simulink model "test_bench"  (Simulink 9.2)
settings: Solver=FixedStepDiscrete  StartTime=0.0  StopTime=inf  FixedStep=t_sample_s  RelTol=1e-3
values from neighbouring files (symbols this model uses):
  f_tp_Hz = 1    [init.m]
  I_gain = [4,4,8,6,11]*1e-2*1    [init.m]
  mpc_flag = 0    [init.m]
  n_akt = 5    [init.m]    (also in postprocess.m)
  offset_q_offline = [266.1,185.3,200.5,240.7,168.1]    [init.m]
  P_gain = [4,6,11,11,10]*1e-2*1    [init.m]
  p_max_bar = 0.7    [init.m]
  pi_flag = 1    [init.m]
  t_sample_s = 1e-3    (= 0.001)    [init.m]
libraries: test_bench_lib x23, etherlab_lib x10, simulink x5, dspsigops x2, pePwmGenerator x1
settings Model: Creator=moritz  LastModifiedBy=entwicklungs-pc  SimulationMode=external  ExtModeTrigDuration=10000  ExtModeArchiveMode=auto  ExtModeArchiveFileName=measurement_data  ExtModeArchiveDirName=./results  ExtModeLogAll=off
settings DataIOCC: LimitDataPoints=off  SaveFormat=Dataset  SignalLoggingSaveFormat=Dataset  SaveOutput=off  SignalLogging=off  SaveTime=off
settings OptimizationCC: BlockReduction=off  ConditionallyExecuteInputs=off  OptimizeBlockIOStorage=off  BufferReuse=off  GlobalBufferReuse=off  ExpressionFolding=off  LocalBlockOutputs=off  LifeSpan=auto  OptimizeDataStoreBuffers=off  BusAssignmentInplaceUpdate=off
settings DebuggingCC: UnderspecifiedInitializationDetection=Simplified  MergeDetectMultiDrivingBlocksExec=error  FcnCallInpInsideContextMsg=error  StateNameClashWarn=none  SFUnexpectedBacktrackingDiag=error  SFNoUnconditionalDefaultTransitionDiag=error  SFExecutionAtInitializationDiag=warning
settings HardwareCC: ProdBitPerPointer=64  ProdBitPerSizeT=64  ProdBitPerPtrDiffT=64  ProdLargestAtomicFloat=Float  ProdIntDivRoundTo=Zero  ProdEndianess=LittleEndian  ProdWordSize=64  ProdHWDeviceType=Intel->x86-64 (Windows64)
settings ModelReferenceCC: PropagateSignalLabelsOutOfModel=on
settings RTWCC: SystemTargetFile=etherlab.tlc  TemplateMakefile=etherlab_hrt.tmf  Description=EtherLab PREEMT_RT Real-Time Target
settings CodeAppCC: StateflowObjectComments=off
settings STFCustomTargetCC: TargetLangStandard=C99 (ISO)  ModelReferenceCompliant=off  SystemTargetFile=etherlab.tlc
settings GRTTargetCC: TargetLangStandard=C99 (ISO)  ModelReferenceCompliant=off  ParMdlRefBuildCompliant=off  CompOptLevelCompliant=off  ConcurrentExecutionCompliant=off  GeneratePreprocessorConditionals=Use local settings  MatFileLogging=off  CPPClassGenCompliant=off  UseToolchainInfoCompliant=off  ExtMode=on  ExtModeStaticAlloc=on  ExtModeStaticAllocSize=50000000  ExtModeMexArgs='130.75.144.164' 0 17725  RTWCAPISignals=on  RTWCAPIParams=on
settings CustomProperty: DataType=int32  Value=2
settings ConfigComp: CovMetricSettings=dwe  CovHtmlReporting=off  CovSaveCumulativeToWorkspaceVar=off  CovSaveSingleToWorkspaceVar=off  CovExternalEMLEnable=on

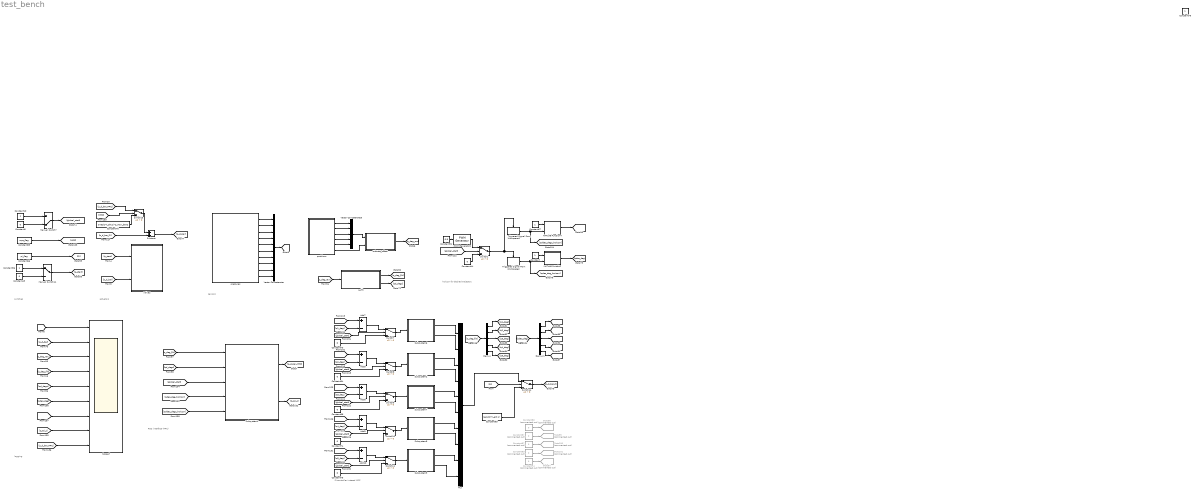
== system test_bench ==
  note: sensors
  note: actuators
  note: logging
  note: switches
  note: ROS interface (MPC)
  note: horizon for desired trajectory
  note: PI-controller instead MPC
  Add{5,7..10} (5 alike) : Sum  Inputs=+-
  Constant{,10,36,67} (4 alike) : Constant  SampleTime=t_sample_s
  Constant{5,43,64,68,73..75} (7 alike) : Constant  Value=0  SampleTime=t_sample_s
  Constant44 : Constant  Value=0  SampleTime=1e-3
  Constant51 : Constant  Value=0.5  SampleTime=t_sample_s
  Constant65 : Constant  Value=zeros(2*n_akt,1)  SampleTime=t_sample_s
  Constant66 : Constant  Value=pi_flag  SampleTime=t_sample_s
  Constant76 : Constant  Value=ones(2*n_akt,1)*p_max_bar/2  SampleTime=t_sample_s
  Constant78 : Constant
  Constant{80..84} (5 alike) : Constant  Commented=on  Value=0
  Constant85 : Constant  Value=mpc_flag  SampleTime=t_sample_s
  Demux : Demux  Outputs=5
  Demux1 : Demux  Outputs=5
  Goto100 : Goto  Commented=on  GotoTag=q3des_deg
  Goto101 : Goto  Commented=on  GotoTag=q4des_deg
  Goto97 : Goto  Commented=on  GotoTag=q5des_deg
  Goto98 : Goto  Commented=on  GotoTag=q1des_deg
  Goto99 : Goto  Commented=on  GotoTag=q2des_deg
  MATLAB Function : MATLAB Function  TreatAsAtomicUnit=on
  MATLAB Function4 : MATLAB Function  TreatAsAtomicUnit=on
  Manual Switch11 : ManualSwitch
  Manual Switch7 : ManualSwitch  CurrentSetting=0
  Mux : Mux  Inputs=10
  PWM Generator2 : pePwmGenerator/PWM Generator  CarrCount=Up  Tper=t_sample_MPC_s  Ts=t_sample_s
  Scope7 : Scope  NumInputPorts=9
  Subsystem2 : Subsystem
  Subsystem4 : Subsystem
  Subsystem6 : Subsystem
  Subsystem7 : Subsystem
  Subsystem8 : Subsystem
  Subsystem9 : Subsystem
  Subtract : Sum
  Switch{1,7..11,13..14} (8 alike) : Switch  Criteria=u2 > Threshold
  Triggered Signal From Workspace1 : dspsigops/Triggered Signal From Workspace  Signal=Qd_total  TriggerType=Rising edge  ic=0  SamplesPerFrame=1  OutputAfterFinalValue=Setting to zero  OutputFrames=off
      settings: SourceProductName=DSP System Toolbox  SourceProductBaseCode=DS
  Triggered Signal From Workspace2 : dspsigops/Triggered Signal From Workspace  Signal=Q_total  TriggerType=Rising edge  ic=0  SamplesPerFrame=1  OutputAfterFinalValue=Setting to zero  OutputFrames=off
      settings: SourceProductName=DSP System Toolbox  SourceProductBaseCode=DS
  Vector Concatenate : Concatenate  NumInputs=10
  Vector Concatenate3 : Concatenate  NumInputs=5
  positions : Subsystem
  pressures : Subsystem
  q_filt : Subsystem
  subtract_offset : MATLAB Function  TreatAsAtomicUnit=on
  "valves " : Subsystem
  wires:
  pressures/3("p21_bar ") -> Vector Concatenate/3
  pressures/4(p22_bar) -> Vector Concatenate/4
  pressures/1("p11_bar ") -> Vector Concatenate/1
  pressures/2(p12_bar) -> Vector Concatenate/2
  pressures/5(p31_bar) -> Vector Concatenate/5
  pressures/6(p32_bar) -> Vector Concatenate/6
  pressures/7(p41_bar) -> Vector Concatenate/7
  pressures/8(p42_bar) -> Vector Concatenate/8
  pressures/9(p51_bar) -> Vector Concatenate/9
  pressures/10(p52_bar) -> Vector Concatenate/10
  [p_d_bar] -> Scope7/2  "p_d_bar"
  Vector Concatenate/1 -> [p_bar]
  positions/1(q1_deg_raw) -> Vector Concatenate3/1
  positions/2(q2_deg_raw) -> Vector Concatenate3/2
  positions/3(q3_deg_raw) -> Vector Concatenate3/3
  positions/4(q4_deg_raw) -> Vector Concatenate3/4
  positions/5(q5_deg_raw) -> Vector Concatenate3/5
  Vector Concatenate3/1 -> subtract_offset/1("q_deg_raw ")
  subtract_offset/1(q_deg_raw) -> [q_deg_raw]
  [p_start] -> "valves "/1(p_start)
  [p_d_bar] -> "valves "/2(p_d_bar)
  [qd_degs] -> Scope7/5  "qd_degs"
  [p_bar] -> Scope7/1  "p_bar"
  [q_deg_raw] -> Scope7/3  "q_deg_raw"
  q_filt/2(qd_degs) -> [qd_degs]
  q_filt/1(q_deg_filt) -> [q_deg_filt]
  [q_deg_filt] -> Scope7/4  "q_deg_filt"
  [q_deg_raw] -> q_filt/1(q_deg_raw)
  [qd_degs] -> Subsystem4/2("qd_degs ")  "qd_degs"
  [q_deg_filt] -> Subsystem4/1(q_deg_filt)  "q_deg_filt"
  [qdes_deg] -> Scope7/6  "qdes_deg"
  Triggered Signal From Workspace2/1 -> [qdes_deg_horizon], MATLAB Function/2(u)
  MATLAB Function/1(y) -> [qdes_deg]
  Constant/1 -> MATLAB Function/1(idx)
  PWM Generator2/1 -> Switch1/1
  Constant51/1 -> PWM Generator2/1
  [global_start] -> Switch1/2
  Switch1/1 -> Triggered Signal From Workspace1/Trigger, Triggered Signal From Workspace2/Trigger  "start_int"
  Constant44/1 -> Switch1/3
  [global_start] -> Subsystem4/3(global_control_start)
  [qdes_deg_horizon] -> Subsystem4/4(qdes_deg_horizon)
  Constant5/1 -> Manual Switch7/2
  Constant10/1 -> Manual Switch7/1
  Manual Switch7/1 -> [global_start]
  Manual Switch11/1 -> [p_start]
  Constant36/1 -> Manual Switch11/1
  Constant43/1 -> Manual Switch11/2
  Subsystem4/1(p_d_bar) -> [p_d_bar_MPC]
  Subtract/1 -> [p_d_bar]
  [p_d_bar_MPC] -> Switch13/1
  positions/6("q_offset ") -> subtract_offset/2(q_offset)
  Demux/5 -> [q5_deg]
  Subsystem9/2(pi2_d_bar) -> Mux/10
  Demux/1 -> [q1_deg]
  Switch14/1 -> [p_d_bar_PI]
  Demux/3 -> [q3_deg]
  [q_deg_filt] -> Demux/1
  Demux/4 -> [q4_deg]
  Demux/2 -> [q2_deg]
  Mux/1 -> Switch14/1
  Demux1/2 -> [q2des_deg]
  Demux1/4 -> [q4des_deg]
  [qdes_deg] -> Demux1/1
  Demux1/3 -> [q3des_deg]
  Demux1/1 -> [q1des_deg]
  Demux1/5 -> [q5des_deg]
  Constant65/1 -> Switch14/3
  [p_d_bar_PI] -> Subtract/2
  Constant73/1 -> Switch7/3
  Switch7/1 -> Subsystem6/1(e_deg)
  Add7/1 -> Switch7/1
  [global_start] -> Switch7/2
  [q1_deg] -> Add7/2
  [q1des_deg] -> Add7/1
  Subsystem6/2(pi2_d_bar) -> Mux/2
  Subsystem6/1(pi1_d_bar) -> Mux/1
  Subsystem2/1(pi1_d_bar) -> Mux/3
  Subsystem2/2(pi2_d_bar) -> Mux/4
  [q2des_deg] -> Add5/1
  [q2_deg] -> Add5/2
  [global_start] -> Switch8/2
  Add5/1 -> Switch8/1
  Switch8/1 -> Subsystem2/1(e_deg)
  Constant64/1 -> Switch8/3
  Constant68/1 -> Switch9/3
  Switch9/1 -> Subsystem7/1(e_deg)
  Add8/1 -> Switch9/1
  [global_start] -> Switch9/2
  [q3_deg] -> Add8/2
  [q3des_deg] -> Add8/1
  Subsystem7/2(pi2_d_bar) -> Mux/6
  Subsystem7/1(pi1_d_bar) -> Mux/5
  Subsystem8/1(pi1_d_bar) -> Mux/7
  Subsystem8/2(pi2_d_bar) -> Mux/8
  [q4des_deg] -> Add9/1
  [q4_deg] -> Add9/2
  [global_start] -> Switch10/2
  Add9/1 -> Switch10/1
  Switch10/1 -> Subsystem8/1(e_deg)
  Constant74/1 -> Switch10/3
  Constant75/1 -> Switch11/3
  Switch11/1 -> Subsystem9/1(e_deg)
  Add10/1 -> Switch11/1
  [global_start] -> Switch11/2
  [q5_deg] -> Add10/2
  [q5des_deg] -> Add10/1
  Subsystem9/1(pi1_d_bar) -> Mux/9
  Switch13/1 -> Subtract/1  "start_int"
  Constant76/1 -> Switch13/3
  Constant80/1 -> Goto98/1
  Constant81/1 -> Goto99/1
  Constant82/1 -> Goto100/1
  Constant83/1 -> Goto101/1
  Constant84/1 -> Goto97/1
  Subsystem4/2(t_sol_s) -> [t_sol_s]
  [t_sol_s] -> Scope7/8  "t_sol_s"
  [PI] -> Switch14/2
  Constant85/1 -> [MPC]
  Constant66/1 -> [PI]
  [p_d_bar_MPC] -> Scope7/9  "p_d_bar_MPC"
  [MPC] -> Switch13/2
  MATLAB Function4/1(y) -> [qddes_degs]
  Triggered Signal From Workspace1/1 -> MATLAB Function4/2(u), [qddes_degs_horizon]
  Constant67/1 -> MATLAB Function4/1(idx)
  [qddes_degs] -> Scope7/7  "qddes_degs"
  [qddes_degs_horizon] -> Subsystem4/5(qddes_degs_horizon)

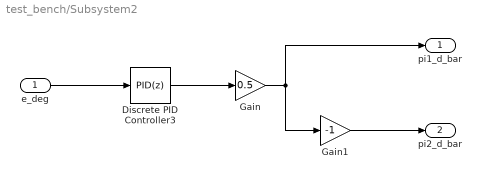
== system test_bench/Subsystem2 ==
  e_deg : Inport
  Discrete PID Controller3 : simulink/Continuous/PID Controller  Controller=PID  Form=Parallel  TimeDomain=Discrete-time  SampleTime=t_sample_s  IntegratorMethod=Forward Euler  FilterMethod=Forward Euler  ControllerParametersSource=internal  P=P_gain(2)  I=I_gain(2)  D=0  UseFilter=on  N=100  TunerSelectOption=Transfer Function Based (PID Tuner App)  InitialConditionSource=internal  InitialConditionForIntegrator=0  InitialConditionForFilter=0  DifferentiatorICPrevScaledInput=0  ExternalReset=none  TrackingMode=off  Kt=1  LimitOutput=on  UpperSaturationLimit=p_max_bar  LowerSaturationLimit=-p_max_bar  LinearizeAsGain=off  AntiWindupMode=back-calculation  Kb=1  POutMin=[]  POutMax=[]  IOutMin=[]  IOutMax=[]  DOutMin=[]  DOutMax=[]  NOutMin=[]  NOutMax=[]  SumOutMin=[]  SumOutMax=[]  SaturationOutMin=[]  SaturationOutMax=[]  PParamMin=[]  PParamMax=[]  IParamMin=[]  IParamMax=[]  DParamMin=[]  DParamMax=[]  NParamMin=[]  NParamMax=[]  KbParamMin=[]  KbParamMax=[]  KtParamMin=[]  KtParamMax=[]  KbOutMin=[]  KbOutMax=[]  KtOutMin=[]  KtOutMax=[]  IntegratorOutMin=[]  IntegratorOutMax=[]  FilterOutMin=[]  FilterOutMax=[]  SumI1OutMin=[]  SumI1OutMax=[]  SumI2OutMin=[]  SumI2OutMax=[]  SumI3OutMin=[]  SumI3OutMax=[]  SumI4OutMin=[]  SumI4OutMax=[]  SumDOutMin=[]  SumDOutMax=[]  DifferentiatorOutMin=[]  DifferentiatorOutMax=[]  FilterDiffOutCoefMin=[]  FilterDiffOutCoefMax=[]  ReciprocalOutMin=[]  ReciprocalOutMax=[]  SumDenOutMin=[]  SumDenOutMax=[]  SumNumOutMin=[]  SumNumOutMax=[]  DivideOutMin=[]  DivideOutMax=[]  IntegratorContinuousStateAttributes=''  IntegratorStateMustResolveToSignalObject=off  IntegratorRTWStateStorageClass=Auto  FilterContinuousStateAttributes=''  FilterStateMustResolveToSignalObject=off  FilterRTWStateStorageClass=Auto  ParallelPVariant=InternalParameters  IdealPVariant=Disabled  IVariant=InternalParameters  DVariant=InternalParameters  IntegratorVariant=Discrete  SatVariant=Enabled  AWVariant=BackCalculation  PCopyVariant=Disabled  TRVariant=Disabled  FdbkBlocksVariant=Forward  IdealPFdbkVariant=Disabled  SatFdbkVariant=Disabled  DerivativeFilterVariant=ForwardEulerFilter  NVariant=InternalParameters  NCopyVariant=Disabled  FilterICVariant=InternalICsFilter  IntegratorICVariant=InternalICs  ExternalResetVariant=Disabled  TRSumVariant=Passthrough  SumFdbkVariant=Disabled  SumVariant=Sum_PID
  Gain : Gain  Gain=0.5
  Gain1 : Gain  Gain=-1
  pi1_d_bar : Outport
  pi2_d_bar : Outport  Port=2
  wires:
  Discrete PID Controller3/1 -> Gain/1
  Gain/1 -> Gain1/1, pi1_d_bar/1
  e_deg/1 -> Discrete PID Controller3/1
  Gain1/1 -> pi2_d_bar/1

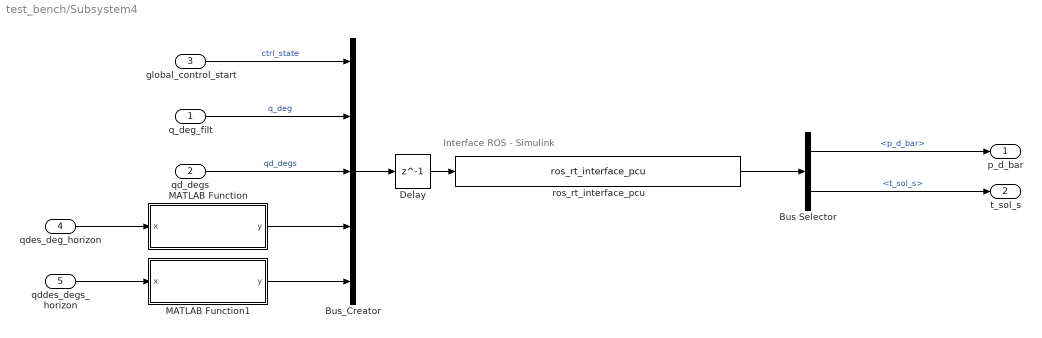
== system test_bench/Subsystem4 ==
  note: Interface ROS - Simulink
  q_deg_filt : Inport
  "qd_degs " : Inport  Port=2
  global_control_start : Inport  Port=3
  qdes_deg_horizon : Inport  Port=4
  qddes_degs_horizon : Inport  Port=5
  Bus Selector : BusSelector  OutputSignals=p_d_bar,t_sol_s
  Bus_Creator : BusCreator  Inputs=5
  Delay : Delay  DelayLength=1  SampleTime=t_sample_s
  MATLAB Function : MATLAB Function  TreatAsAtomicUnit=on  SystemSampleTime=t_sample_s
  MATLAB Function1 : MATLAB Function  TreatAsAtomicUnit=on  SystemSampleTime=t_sample_s
  ros_rt_interface_pcu : S-Function  FunctionName=ros_rt_interface_pcu  SFunctionDeploymentMode=off  EnableBusSupport=off  mask(Legacy Function){SFunctionSpec=void SL_io_func(SL_OUT_type u1[1], SL_IN_type y1[1]), ShowSpec=on}
      mask prompts: ShowSpec "Display function specification"
      mask help:
      | This block allows you to call the legacy functions specified by the following Legacy Code Tool definition:
      | def.SFunctionName = 'ros_rt_interface_pcu';
      | def.OutputFcnSpec = 'void SL_io_func(SL_OUT_type u1[1], SL_IN_type y1[1])';
      | def.StartFcnSpec = 'void SL_start_func()';
      | def.TerminateFcnSpec = 'void SL_terminate_func()';
      | def.HeaderFiles = {'SL_func.h'};
      | def.SourceFiles = {'../ros_rt_interface/ros_rt_core/SL_func_dummy.cpp'};
      | def.TargetLibFiles = {'libros_sl_interface.so'};
      | def.IncPaths = {'../ros_rt_interface/ros_rt_core'};
      mask Help: <p>This block was generated automatically by the Legacy Code Tool. For detailed help on this tool, call<a href="matlab:legacy_code('help')"> legacy_code('help')</a>.</p>
      mask Callback ShowSpec:
      | if strcmp(get_param(gcbh, 'ShowSpec'), 'on')
      |   set_param(gcbh, 'MaskDisplay', sprintf('fprintf(''%s'');', get_param(gcbh, 'SFunctionSpec')));
      | else
      |   set_param(gcbh, 'MaskDisplay', sprintf('fprintf(''%s'');', get_param(gcbh, 'FunctionName')));
      | end
      mask Display: fprintf('void SL_io_func(SL_OUT_type u1[1], SL_IN_type y1[1])');
  p_d_bar : Outport
  t_sol_s : Outport  Port=2
  wires:
  Delay/1 -> ros_rt_interface_pcu/1
  Bus Selector/1 -> p_d_bar/1  "<p_d_bar>"
  Bus_Creator/1 -> Delay/1
  global_control_start/1 -> Bus_Creator/1  "ctrl_state"
  "qd_degs "/1 -> Bus_Creator/3  "qd_degs"
  q_deg_filt/1 -> Bus_Creator/2  "q_deg"
  qdes_deg_horizon/1 -> MATLAB Function/1(x)
  MATLAB Function/1(y) -> Bus_Creator/4
  ros_rt_interface_pcu/1 -> Bus Selector/1
  Bus Selector/2 -> t_sol_s/1  "<t_sol_s>"
  qddes_degs_horizon/1 -> MATLAB Function1/1(x)
  MATLAB Function1/1(y) -> Bus_Creator/5

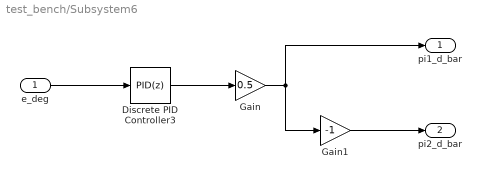
== system test_bench/Subsystem6 ==
  e_deg : Inport
  Discrete PID Controller3 : simulink/Continuous/PID Controller  Controller=PID  Form=Parallel  TimeDomain=Discrete-time  SampleTime=t_sample_s  IntegratorMethod=Forward Euler  FilterMethod=Forward Euler  ControllerParametersSource=internal  P=P_gain(1)  I=I_gain(1)  D=0  UseFilter=on  N=100  TunerSelectOption=Transfer Function Based (PID Tuner App)  InitialConditionSource=internal  InitialConditionForIntegrator=0  InitialConditionForFilter=0  DifferentiatorICPrevScaledInput=0  ExternalReset=none  TrackingMode=off  Kt=1  LimitOutput=on  UpperSaturationLimit=p_max_bar  LowerSaturationLimit=-p_max_bar  LinearizeAsGain=off  AntiWindupMode=back-calculation  Kb=1  POutMin=[]  POutMax=[]  IOutMin=[]  IOutMax=[]  DOutMin=[]  DOutMax=[]  NOutMin=[]  NOutMax=[]  SumOutMin=[]  SumOutMax=[]  SaturationOutMin=[]  SaturationOutMax=[]  PParamMin=[]  PParamMax=[]  IParamMin=[]  IParamMax=[]  DParamMin=[]  DParamMax=[]  NParamMin=[]  NParamMax=[]  KbParamMin=[]  KbParamMax=[]  KtParamMin=[]  KtParamMax=[]  KbOutMin=[]  KbOutMax=[]  KtOutMin=[]  KtOutMax=[]  IntegratorOutMin=[]  IntegratorOutMax=[]  FilterOutMin=[]  FilterOutMax=[]  SumI1OutMin=[]  SumI1OutMax=[]  SumI2OutMin=[]  SumI2OutMax=[]  SumI3OutMin=[]  SumI3OutMax=[]  SumI4OutMin=[]  SumI4OutMax=[]  SumDOutMin=[]  SumDOutMax=[]  DifferentiatorOutMin=[]  DifferentiatorOutMax=[]  FilterDiffOutCoefMin=[]  FilterDiffOutCoefMax=[]  ReciprocalOutMin=[]  ReciprocalOutMax=[]  SumDenOutMin=[]  SumDenOutMax=[]  SumNumOutMin=[]  SumNumOutMax=[]  DivideOutMin=[]  DivideOutMax=[]  IntegratorContinuousStateAttributes=''  IntegratorStateMustResolveToSignalObject=off  IntegratorRTWStateStorageClass=Auto  FilterContinuousStateAttributes=''  FilterStateMustResolveToSignalObject=off  FilterRTWStateStorageClass=Auto  ParallelPVariant=InternalParameters  IdealPVariant=Disabled  IVariant=InternalParameters  DVariant=InternalParameters  IntegratorVariant=Discrete  SatVariant=Enabled  AWVariant=BackCalculation  PCopyVariant=Disabled  TRVariant=Disabled  FdbkBlocksVariant=Forward  IdealPFdbkVariant=Disabled  SatFdbkVariant=Disabled  DerivativeFilterVariant=ForwardEulerFilter  NVariant=InternalParameters  NCopyVariant=Disabled  FilterICVariant=InternalICsFilter  IntegratorICVariant=InternalICs  ExternalResetVariant=Disabled  TRSumVariant=Passthrough  SumFdbkVariant=Disabled  SumVariant=Sum_PID
  Gain : Gain  Gain=0.5
  Gain1 : Gain  Gain=-1
  pi1_d_bar : Outport
  pi2_d_bar : Outport  Port=2
  wires:
  Gain1/1 -> pi2_d_bar/1
  e_deg/1 -> Discrete PID Controller3/1
  Gain/1 -> pi1_d_bar/1, Gain1/1
  Discrete PID Controller3/1 -> Gain/1

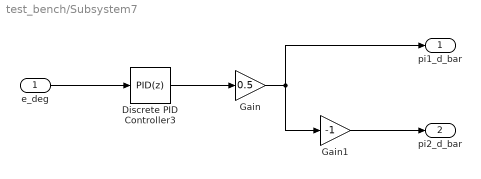
== system test_bench/Subsystem7 ==
  e_deg : Inport
  Discrete PID Controller3 : simulink/Continuous/PID Controller  Controller=PID  Form=Parallel  TimeDomain=Discrete-time  SampleTime=t_sample_s  IntegratorMethod=Forward Euler  FilterMethod=Forward Euler  ControllerParametersSource=internal  P=P_gain(3)  I=I_gain(3)  D=0  UseFilter=on  N=100  TunerSelectOption=Transfer Function Based (PID Tuner App)  InitialConditionSource=internal  InitialConditionForIntegrator=0  InitialConditionForFilter=0  DifferentiatorICPrevScaledInput=0  ExternalReset=none  TrackingMode=off  Kt=1  LimitOutput=on  UpperSaturationLimit=p_max_bar  LowerSaturationLimit=-p_max_bar  LinearizeAsGain=off  AntiWindupMode=back-calculation  Kb=1  POutMin=[]  POutMax=[]  IOutMin=[]  IOutMax=[]  DOutMin=[]  DOutMax=[]  NOutMin=[]  NOutMax=[]  SumOutMin=[]  SumOutMax=[]  SaturationOutMin=[]  SaturationOutMax=[]  PParamMin=[]  PParamMax=[]  IParamMin=[]  IParamMax=[]  DParamMin=[]  DParamMax=[]  NParamMin=[]  NParamMax=[]  KbParamMin=[]  KbParamMax=[]  KtParamMin=[]  KtParamMax=[]  KbOutMin=[]  KbOutMax=[]  KtOutMin=[]  KtOutMax=[]  IntegratorOutMin=[]  IntegratorOutMax=[]  FilterOutMin=[]  FilterOutMax=[]  SumI1OutMin=[]  SumI1OutMax=[]  SumI2OutMin=[]  SumI2OutMax=[]  SumI3OutMin=[]  SumI3OutMax=[]  SumI4OutMin=[]  SumI4OutMax=[]  SumDOutMin=[]  SumDOutMax=[]  DifferentiatorOutMin=[]  DifferentiatorOutMax=[]  FilterDiffOutCoefMin=[]  FilterDiffOutCoefMax=[]  ReciprocalOutMin=[]  ReciprocalOutMax=[]  SumDenOutMin=[]  SumDenOutMax=[]  SumNumOutMin=[]  SumNumOutMax=[]  DivideOutMin=[]  DivideOutMax=[]  IntegratorContinuousStateAttributes=''  IntegratorStateMustResolveToSignalObject=off  IntegratorRTWStateStorageClass=Auto  FilterContinuousStateAttributes=''  FilterStateMustResolveToSignalObject=off  FilterRTWStateStorageClass=Auto  ParallelPVariant=InternalParameters  IdealPVariant=Disabled  IVariant=InternalParameters  DVariant=InternalParameters  IntegratorVariant=Discrete  SatVariant=Enabled  AWVariant=BackCalculation  PCopyVariant=Disabled  TRVariant=Disabled  FdbkBlocksVariant=Forward  IdealPFdbkVariant=Disabled  SatFdbkVariant=Disabled  DerivativeFilterVariant=ForwardEulerFilter  NVariant=InternalParameters  NCopyVariant=Disabled  FilterICVariant=InternalICsFilter  IntegratorICVariant=InternalICs  ExternalResetVariant=Disabled  TRSumVariant=Passthrough  SumFdbkVariant=Disabled  SumVariant=Sum_PID
  Gain : Gain  Gain=0.5
  Gain1 : Gain  Gain=-1
  pi1_d_bar : Outport
  pi2_d_bar : Outport  Port=2
  wires:
  Gain1/1 -> pi2_d_bar/1
  e_deg/1 -> Discrete PID Controller3/1
  Gain/1 -> pi1_d_bar/1, Gain1/1
  Discrete PID Controller3/1 -> Gain/1

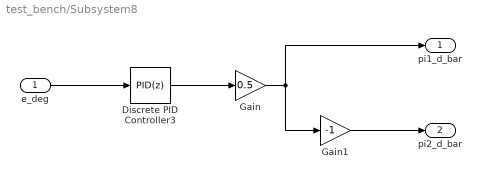
== system test_bench/Subsystem8 ==
  e_deg : Inport
  Discrete PID Controller3 : simulink/Continuous/PID Controller  Controller=PID  Form=Parallel  TimeDomain=Discrete-time  SampleTime=t_sample_s  IntegratorMethod=Forward Euler  FilterMethod=Forward Euler  ControllerParametersSource=internal  P=P_gain(4)  I=I_gain(4)  D=0  UseFilter=on  N=100  TunerSelectOption=Transfer Function Based (PID Tuner App)  InitialConditionSource=internal  InitialConditionForIntegrator=0  InitialConditionForFilter=0  DifferentiatorICPrevScaledInput=0  ExternalReset=none  TrackingMode=off  Kt=1  LimitOutput=on  UpperSaturationLimit=p_max_bar  LowerSaturationLimit=-p_max_bar  LinearizeAsGain=off  AntiWindupMode=back-calculation  Kb=1  POutMin=[]  POutMax=[]  IOutMin=[]  IOutMax=[]  DOutMin=[]  DOutMax=[]  NOutMin=[]  NOutMax=[]  SumOutMin=[]  SumOutMax=[]  SaturationOutMin=[]  SaturationOutMax=[]  PParamMin=[]  PParamMax=[]  IParamMin=[]  IParamMax=[]  DParamMin=[]  DParamMax=[]  NParamMin=[]  NParamMax=[]  KbParamMin=[]  KbParamMax=[]  KtParamMin=[]  KtParamMax=[]  KbOutMin=[]  KbOutMax=[]  KtOutMin=[]  KtOutMax=[]  IntegratorOutMin=[]  IntegratorOutMax=[]  FilterOutMin=[]  FilterOutMax=[]  SumI1OutMin=[]  SumI1OutMax=[]  SumI2OutMin=[]  SumI2OutMax=[]  SumI3OutMin=[]  SumI3OutMax=[]  SumI4OutMin=[]  SumI4OutMax=[]  SumDOutMin=[]  SumDOutMax=[]  DifferentiatorOutMin=[]  DifferentiatorOutMax=[]  FilterDiffOutCoefMin=[]  FilterDiffOutCoefMax=[]  ReciprocalOutMin=[]  ReciprocalOutMax=[]  SumDenOutMin=[]  SumDenOutMax=[]  SumNumOutMin=[]  SumNumOutMax=[]  DivideOutMin=[]  DivideOutMax=[]  IntegratorContinuousStateAttributes=''  IntegratorStateMustResolveToSignalObject=off  IntegratorRTWStateStorageClass=Auto  FilterContinuousStateAttributes=''  FilterStateMustResolveToSignalObject=off  FilterRTWStateStorageClass=Auto  ParallelPVariant=InternalParameters  IdealPVariant=Disabled  IVariant=InternalParameters  DVariant=InternalParameters  IntegratorVariant=Discrete  SatVariant=Enabled  AWVariant=BackCalculation  PCopyVariant=Disabled  TRVariant=Disabled  FdbkBlocksVariant=Forward  IdealPFdbkVariant=Disabled  SatFdbkVariant=Disabled  DerivativeFilterVariant=ForwardEulerFilter  NVariant=InternalParameters  NCopyVariant=Disabled  FilterICVariant=InternalICsFilter  IntegratorICVariant=InternalICs  ExternalResetVariant=Disabled  TRSumVariant=Passthrough  SumFdbkVariant=Disabled  SumVariant=Sum_PID
  Gain : Gain  Gain=0.5
  Gain1 : Gain  Gain=-1
  pi1_d_bar : Outport
  pi2_d_bar : Outport  Port=2
  wires:
  Discrete PID Controller3/1 -> Gain/1
  Gain/1 -> Gain1/1, pi1_d_bar/1
  e_deg/1 -> Discrete PID Controller3/1
  Gain1/1 -> pi2_d_bar/1

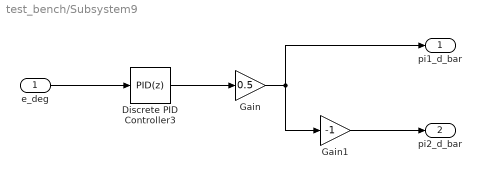
== system test_bench/Subsystem9 ==
  e_deg : Inport
  Discrete PID Controller3 : simulink/Continuous/PID Controller  Controller=PID  Form=Parallel  TimeDomain=Discrete-time  SampleTime=t_sample_s  IntegratorMethod=Forward Euler  FilterMethod=Forward Euler  ControllerParametersSource=internal  P=P_gain(5)  I=I_gain(5)  D=0  UseFilter=on  N=100  TunerSelectOption=Transfer Function Based (PID Tuner App)  InitialConditionSource=internal  InitialConditionForIntegrator=0  InitialConditionForFilter=0  DifferentiatorICPrevScaledInput=0  ExternalReset=none  TrackingMode=off  Kt=1  LimitOutput=on  UpperSaturationLimit=p_max_bar  LowerSaturationLimit=-p_max_bar  LinearizeAsGain=off  AntiWindupMode=back-calculation  Kb=1  POutMin=[]  POutMax=[]  IOutMin=[]  IOutMax=[]  DOutMin=[]  DOutMax=[]  NOutMin=[]  NOutMax=[]  SumOutMin=[]  SumOutMax=[]  SaturationOutMin=[]  SaturationOutMax=[]  PParamMin=[]  PParamMax=[]  IParamMin=[]  IParamMax=[]  DParamMin=[]  DParamMax=[]  NParamMin=[]  NParamMax=[]  KbParamMin=[]  KbParamMax=[]  KtParamMin=[]  KtParamMax=[]  KbOutMin=[]  KbOutMax=[]  KtOutMin=[]  KtOutMax=[]  IntegratorOutMin=[]  IntegratorOutMax=[]  FilterOutMin=[]  FilterOutMax=[]  SumI1OutMin=[]  SumI1OutMax=[]  SumI2OutMin=[]  SumI2OutMax=[]  SumI3OutMin=[]  SumI3OutMax=[]  SumI4OutMin=[]  SumI4OutMax=[]  SumDOutMin=[]  SumDOutMax=[]  DifferentiatorOutMin=[]  DifferentiatorOutMax=[]  FilterDiffOutCoefMin=[]  FilterDiffOutCoefMax=[]  ReciprocalOutMin=[]  ReciprocalOutMax=[]  SumDenOutMin=[]  SumDenOutMax=[]  SumNumOutMin=[]  SumNumOutMax=[]  DivideOutMin=[]  DivideOutMax=[]  IntegratorContinuousStateAttributes=''  IntegratorStateMustResolveToSignalObject=off  IntegratorRTWStateStorageClass=Auto  FilterContinuousStateAttributes=''  FilterStateMustResolveToSignalObject=off  FilterRTWStateStorageClass=Auto  ParallelPVariant=InternalParameters  IdealPVariant=Disabled  IVariant=InternalParameters  DVariant=InternalParameters  IntegratorVariant=Discrete  SatVariant=Enabled  AWVariant=BackCalculation  PCopyVariant=Disabled  TRVariant=Disabled  FdbkBlocksVariant=Forward  IdealPFdbkVariant=Disabled  SatFdbkVariant=Disabled  DerivativeFilterVariant=ForwardEulerFilter  NVariant=InternalParameters  NCopyVariant=Disabled  FilterICVariant=InternalICsFilter  IntegratorICVariant=InternalICs  ExternalResetVariant=Disabled  TRSumVariant=Passthrough  SumFdbkVariant=Disabled  SumVariant=Sum_PID
  Gain : Gain  Gain=0.5
  Gain1 : Gain  Gain=-1
  pi1_d_bar : Outport
  pi2_d_bar : Outport  Port=2
  wires:
  Gain1/1 -> pi2_d_bar/1
  e_deg/1 -> Discrete PID Controller3/1
  Gain/1 -> pi1_d_bar/1, Gain1/1
  Discrete PID Controller3/1 -> Gain/1

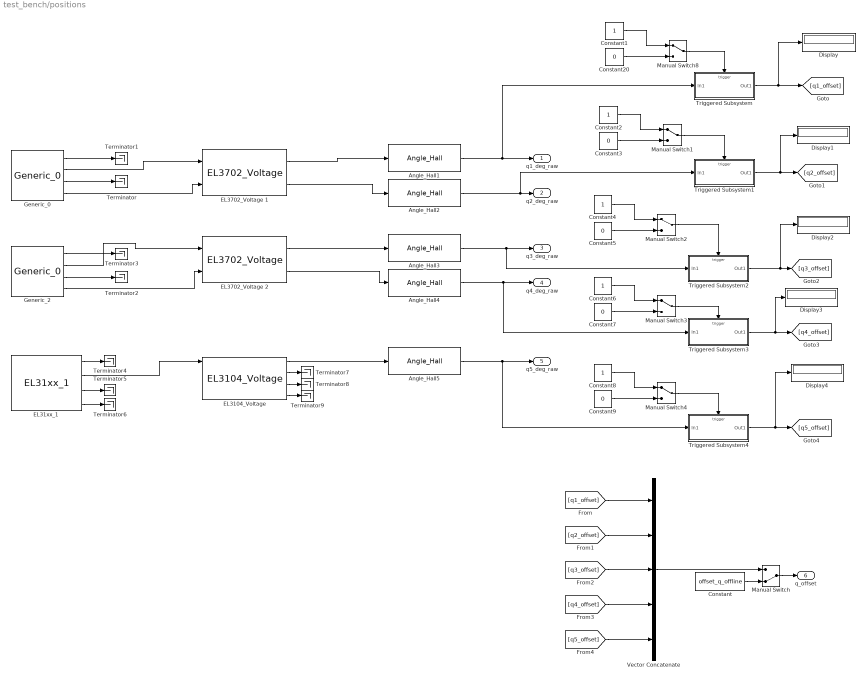
== system test_bench/positions ==
  Angle_Hall{1..5} (5 alike) : test_bench_lib/Angle_Hall  SystemSampleTime=-1
  Constant : Constant  Value=offset_q_offline  SampleTime=t_sample_s
  Constant{1..2,4,6,8} (5 alike) : Constant  SampleTime=t_sample_s
  Constant{3,5,7,9,20} (5 alike) : Constant  Value=0  SampleTime=t_sample_s
  Display{,1..4} (5 alike) : Display
  EL3104_Voltage : test_bench_lib/EL3104_Voltage  SystemSampleTime=-1
  EL31xx_1 : etherlab_lib/EtherCAT/Beckhoff/EL31xx_1  master=0  index=9  model=EL3104  revision=[203436114 1179648]  vector=off  status=off  filter=Off  gain=[]  offset=[]  tau=[]  tsample=t_sample_s  debug=0  dc_mode=Free Run/SM-Synchron  dc_assign_activate=hex2dec('700')  dc_cycle0=[]  dc_cycle0_factor=[]  dc_shift0=[]  dc_shift0_factor=[]  dc_shift0_input=off  dc_cycle1=[]  dc_cycle1_factor=[]  dc_shift1=[]  dc_shift1_factor=[]
      settings: AttributesFormatString=|
      | EL3104
      | M:0 Idx:9
  EL3702_Voltage 1 : test_bench_lib/EL3702_Voltage  SystemSampleTime=-1
  EL3702_Voltage 2 : test_bench_lib/EL3702_Voltage  SystemSampleTime=-1
  Generic_0 : etherlab_lib/EtherCAT/Generic_0  master=0  index=6  rv=slave_el3102  param=[]  tsample=t_sample_s  debug=0
  Generic_2 : etherlab_lib/EtherCAT/Generic_0  master=0  index=7  rv=slave_el3102  param=[]  tsample=t_sample_s  debug=0
  Manual Switch : ManualSwitch  CurrentSetting=0
  Manual Switch{1..4,8} (5 alike) : ManualSwitch
  Terminator{,1..9} (10 alike) : Terminator
  Triggered Subsystem : Subsystem  TreatAsAtomicUnit=on
  Triggered Subsystem1 : Subsystem  TreatAsAtomicUnit=on
  Triggered Subsystem2 : Subsystem  TreatAsAtomicUnit=on
  Triggered Subsystem3 : Subsystem  TreatAsAtomicUnit=on
  Triggered Subsystem4 : Subsystem  TreatAsAtomicUnit=on
  Vector Concatenate : Concatenate  NumInputs=5
  q1_deg_raw : Outport
  q2_deg_raw : Outport  Port=2
  q3_deg_raw : Outport  Port=3
  q4_deg_raw : Outport  Port=4
  q5_deg_raw : Outport  Port=5
  "q_offset " : Outport  Port=6
  wires:
  EL3702_Voltage 1/1 -> Angle_Hall1/1
  Generic_0/4 -> EL3702_Voltage 1/2
  EL3702_Voltage 2/1 -> Angle_Hall3/1
  Generic_2/4 -> EL3702_Voltage 2/2
  EL3104_Voltage/3 -> Terminator8/1
  Generic_0/3 -> Terminator/1
  Generic_0/2 -> EL3702_Voltage 1/1
  EL3702_Voltage 1/2 -> Angle_Hall2/1
  Generic_2/3 -> Terminator2/1
  EL3104_Voltage/2 -> Terminator7/1
  EL3104_Voltage/1 -> Angle_Hall5/1
  EL3702_Voltage 2/2 -> Angle_Hall4/1
  Generic_2/1 -> Terminator3/1
  Generic_0/1 -> Terminator1/1
  Generic_2/2 -> EL3702_Voltage 2/1
  EL3104_Voltage/4 -> Terminator9/1
  EL31xx_1/1 -> Terminator4/1
  EL31xx_1/4 -> Terminator6/1
  EL31xx_1/3 -> Terminator5/1
  EL31xx_1/2 -> EL3104_Voltage/1
  Angle_Hall4/1 -> Triggered Subsystem3/1(In1), q4_deg_raw/1
  Manual Switch4/1 -> Triggered Subsystem4/Trigger
  Angle_Hall1/1 -> Triggered Subsystem/1(In1), q1_deg_raw/1
  Constant1/1 -> Manual Switch8/1
  Manual Switch2/1 -> Triggered Subsystem2/Trigger
  Constant5/1 -> Manual Switch2/2
  Manual Switch8/1 -> Triggered Subsystem/Trigger
  Constant4/1 -> Manual Switch2/1
  Constant9/1 -> Manual Switch4/2
  Constant8/1 -> Manual Switch4/1
  Angle_Hall5/1 -> q5_deg_raw/1, Triggered Subsystem4/1(In1)
  Constant6/1 -> Manual Switch3/1
  Constant7/1 -> Manual Switch3/2
  Angle_Hall3/1 -> Triggered Subsystem2/1(In1), q3_deg_raw/1
  Manual Switch3/1 -> Triggered Subsystem3/Trigger
  Constant20/1 -> Manual Switch8/2
  Constant2/1 -> Manual Switch1/1
  Constant3/1 -> Manual Switch1/2
  Triggered Subsystem/1(Out1) -> Display/1, [q1_offset]
  Manual Switch1/1 -> Triggered Subsystem1/Trigger
  Angle_Hall2/1 -> Triggered Subsystem1/1(In1), q2_deg_raw/1
  [q4_offset] -> Vector Concatenate/4
  [q3_offset] -> Vector Concatenate/3
  [q2_offset] -> Vector Concatenate/2
  Vector Concatenate/1 -> Manual Switch/1
  [q1_offset] -> Vector Concatenate/1
  [q5_offset] -> Vector Concatenate/5
  Manual Switch/1 -> "q_offset "/1
  Constant/1 -> Manual Switch/2
  Triggered Subsystem1/1(Out1) -> Display1/1, [q2_offset]
  Triggered Subsystem2/1(Out1) -> Display2/1, [q3_offset]
  Triggered Subsystem3/1(Out1) -> [q4_offset], Display3/1
  Triggered Subsystem4/1(Out1) -> Display4/1, [q5_offset]

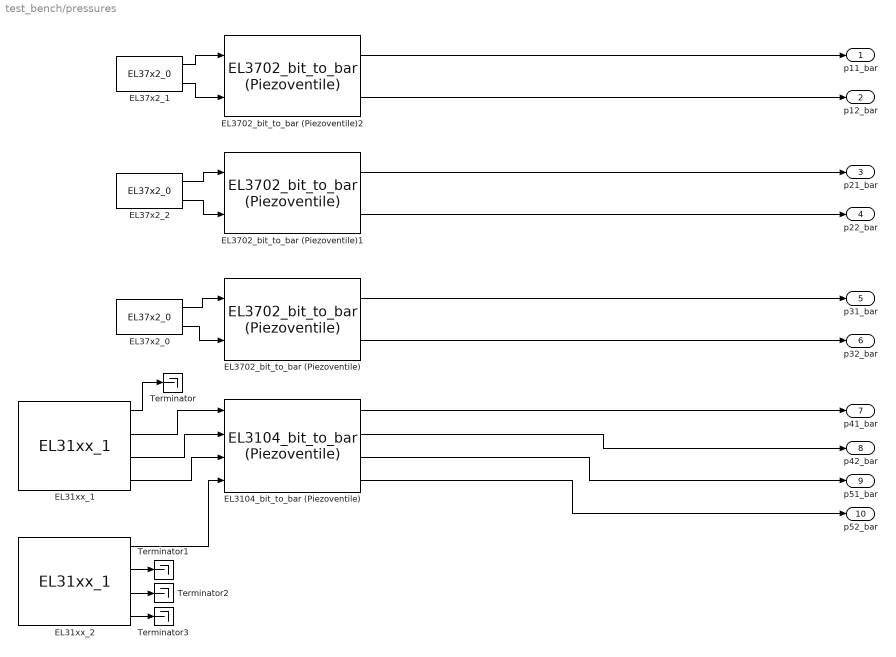
== system test_bench/pressures ==
  EL3104_bit_to_bar (Piezoventile) : test_bench_lib/EL3104_bit_to_bar (Piezoventile)  SystemSampleTime=-1
  EL31xx_1 : etherlab_lib/EtherCAT/Beckhoff/EL31xx_1  master=0  index=8  model=EL3104  revision=[203436114 1179648]  vector=off  status=off  filter=Off  gain=[]  offset=[]  tau=[]  tsample=t_sample_s  debug=0  dc_mode=Free Run/SM-Synchron  dc_assign_activate=hex2dec('700')  dc_cycle0=[]  dc_cycle0_factor=[]  dc_shift0=[]  dc_shift0_factor=[]  dc_shift0_input=off  dc_cycle1=[]  dc_cycle1_factor=[]  dc_shift1=[]  dc_shift1_factor=[]
      settings: AttributesFormatString=|
      | EL3104
      | M:0 Idx:8
  EL31xx_2 : etherlab_lib/EtherCAT/Beckhoff/EL31xx_1  master=0  index=9  model=EL3104  revision=[203436114 1179648]  vector=off  status=off  filter=Off  gain=[]  offset=[]  tau=[]  tsample=t_sample_s  debug=0  dc_mode=Free Run/SM-Synchron  dc_assign_activate=hex2dec('700')  dc_cycle0=[]  dc_cycle0_factor=[]  dc_shift0=[]  dc_shift0_factor=[]  dc_shift0_input=off  dc_cycle1=[]  dc_cycle1_factor=[]  dc_shift1=[]  dc_shift1_factor=[]
      settings: AttributesFormatString=|
      | EL3104
      | M:0 Idx:9
  EL3702_bit_to_bar (Piezoventile) : test_bench_lib/EL3702_bit_to_bar (Piezoventile)  SystemSampleTime=-1
  EL3702_bit_to_bar (Piezoventile)1 : test_bench_lib/EL3702_bit_to_bar (Piezoventile)  SystemSampleTime=-1
  EL3702_bit_to_bar (Piezoventile)2 : test_bench_lib/EL3702_bit_to_bar (Piezoventile)  SystemSampleTime=-1
  EL37x2_0 : etherlab_lib/EtherCAT/Beckhoff/EL37x2_0  master=0  index=5  model=EL3702  revision=[242626642 131072]  one_ch=off  scale=[]  offset=[]  tsample=t_sample_s  debug=0  dc_mode=1  dc_assign_activate=hex2dec('730')  dc_cycle0=0  dc_cycle0_factor="-10     % 10-times OS"  dc_shift0=-10000  dc_shift0_factor=1  dc_shift0_input=off  dc_cycle1=0  dc_cycle1_factor=-1  dc_shift1=0  dc_shift1_factor=0
  EL37x2_1 : etherlab_lib/EtherCAT/Beckhoff/EL37x2_0  master=0  index=3  model=EL3702  revision=[242626642 131072]  one_ch=off  scale=[]  offset=[]  tsample=t_sample_s  debug=0  dc_mode=1  dc_assign_activate=hex2dec('730')  dc_cycle0=0  dc_cycle0_factor="-10     % 10-times OS"  dc_shift0=-10000  dc_shift0_factor=1  dc_shift0_input=off  dc_cycle1=0  dc_cycle1_factor=-1  dc_shift1=0  dc_shift1_factor=0
  EL37x2_2 : etherlab_lib/EtherCAT/Beckhoff/EL37x2_0  master=0  index=4  model=EL3702  revision=[242626642 131072]  one_ch=off  scale=[]  offset=[]  tsample=t_sample_s  debug=0  dc_mode=1  dc_assign_activate=hex2dec('730')  dc_cycle0=0  dc_cycle0_factor="-10     % 10-times OS"  dc_shift0=-10000  dc_shift0_factor=1  dc_shift0_input=off  dc_cycle1=0  dc_cycle1_factor=-1  dc_shift1=0  dc_shift1_factor=0
  Terminator{,1..3} (4 alike) : Terminator
  "p11_bar " : Outport
  p12_bar : Outport  Port=2
  "p21_bar " : Outport  Port=3
  p22_bar : Outport  Port=4
  p31_bar : Outport  Port=5
  p32_bar : Outport  Port=6
  p41_bar : Outport  Port=7
  p42_bar : Outport  Port=8
  p51_bar : Outport  Port=9
  p52_bar : Outport  Port=10
  wires:
  EL37x2_0/1 -> EL3702_bit_to_bar (Piezoventile)/1
  EL3702_bit_to_bar (Piezoventile)/2 -> p32_bar/1
  EL3702_bit_to_bar (Piezoventile)/1 -> p31_bar/1
  EL37x2_0/2 -> EL3702_bit_to_bar (Piezoventile)/2
  EL37x2_1/2 -> EL3702_bit_to_bar (Piezoventile)2/2
  EL37x2_1/1 -> EL3702_bit_to_bar (Piezoventile)2/1
  EL3702_bit_to_bar (Piezoventile)1/2 -> p22_bar/1
  EL37x2_2/2 -> EL3702_bit_to_bar (Piezoventile)1/2
  EL37x2_2/1 -> EL3702_bit_to_bar (Piezoventile)1/1
  EL3702_bit_to_bar (Piezoventile)1/1 -> "p21_bar "/1
  EL3702_bit_to_bar (Piezoventile)2/1 -> "p11_bar "/1
  EL3702_bit_to_bar (Piezoventile)2/2 -> p12_bar/1
  EL3104_bit_to_bar (Piezoventile)/2 -> p42_bar/1
  EL3104_bit_to_bar (Piezoventile)/1 -> p41_bar/1
  EL3104_bit_to_bar (Piezoventile)/4 -> p52_bar/1
  EL3104_bit_to_bar (Piezoventile)/3 -> p51_bar/1
  EL31xx_1/2 -> EL3104_bit_to_bar (Piezoventile)/1
  EL31xx_1/3 -> EL3104_bit_to_bar (Piezoventile)/2
  EL31xx_1/4 -> EL3104_bit_to_bar (Piezoventile)/3
  EL31xx_2/1 -> EL3104_bit_to_bar (Piezoventile)/4
  EL31xx_1/1 -> Terminator/1
  EL31xx_2/2 -> Terminator1/1
  EL31xx_2/3 -> Terminator2/1
  EL31xx_2/4 -> Terminator3/1

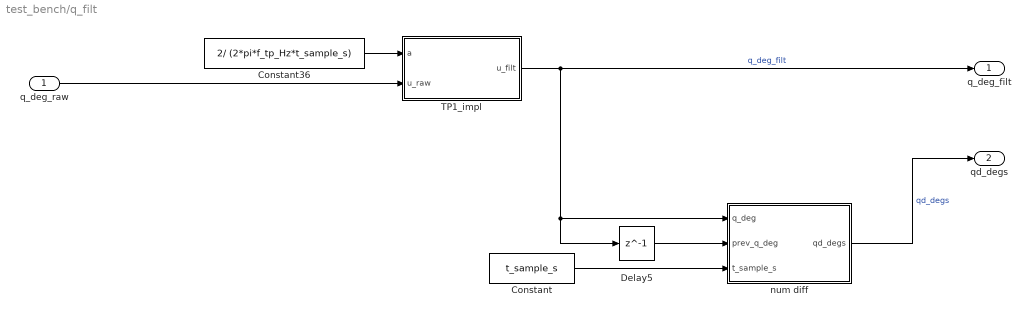
== system test_bench/q_filt ==
  q_deg_raw : Inport
  Constant : Constant  Value=t_sample_s  SampleTime=t_sample_s
  Constant36 : Constant  Value=2/ (2*pi*f_tp_Hz*t_sample_s)  SampleTime=t_sample_s
  Delay5 : Delay  DelayLength=1  InitialCondition=zeros(1,5)  SampleTime=t_sample_s
  TP1_impl : Subsystem
  num diff : MATLAB Function  TreatAsAtomicUnit=on
  q_deg_filt : Outport
  qd_degs : Outport  Port=2
  wires:
  Constant36/1 -> TP1_impl/1(a)
  Constant/1 -> num diff/3(t_sample_s)
  q_deg_raw/1 -> TP1_impl/2(u_raw)
  Delay5/1 -> num diff/2(prev_q_deg)
  TP1_impl/1(u_filt) -> q_deg_filt/1, Delay5/1, num diff/1(q_deg)  "q_deg_filt"
  num diff/1(qd_degs) -> qd_degs/1  "qd_degs"

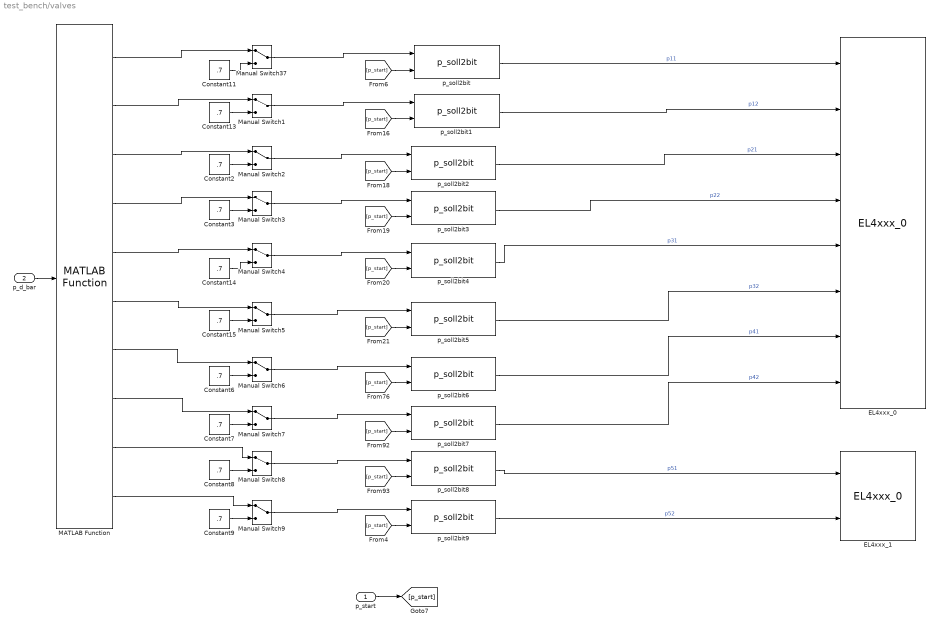
== system test_bench/valves  ==
  p_start : Inport
  p_d_bar : Inport  Port=2
  Constant{2..3,6..9,11,13..15} (10 alike) : Constant  Value=.7  SampleTime=t_sample_s
  EL4xxx_0 : etherlab_lib/EtherCAT/Beckhoff/EL4xxx_0  master=0  index=10  model=EL4008  revision=[262680658 1245184]  vector=off  scale=[]  tsample=t_sample_s  debug=0  dc_mode=Free Run  dc_assign_activate=hex2dec('700')  dc_cycle0=0  dc_cycle0_factor=1  dc_shift0=0  dc_shift0_factor=0  dc_shift0_input=off  dc_cycle1=0  dc_cycle1_factor=1  dc_shift1=10000  dc_shift1_factor=0
  EL4xxx_1 : etherlab_lib/EtherCAT/Beckhoff/EL4xxx_0  master=0  index=11  model=EL4102  revision=[268841042 66715648]  vector=off  scale=[]  tsample=t_sample_s  debug=0  dc_mode=Free Run  dc_assign_activate=hex2dec('700')  dc_cycle0=0  dc_cycle0_factor=1  dc_shift0=0  dc_shift0_factor=0  dc_shift0_input=off  dc_cycle1=0  dc_cycle1_factor=1  dc_shift1=10000  dc_shift1_factor=0
  MATLAB Function : test_bench_lib/MATLAB Function  SystemSampleTime=-1
  Manual Switch{1..9,37} (10 alike) : ManualSwitch
  p_soll2bit{,1..9} (10 alike) : test_bench_lib/p_soll2bit  SystemSampleTime=-1
  wires:
  [p_start] -> p_soll2bit3/2
  p_soll2bit9/1 -> EL4xxx_1/2  "p52"
  p_soll2bit7/1 -> EL4xxx_0/8  "p42"
  p_soll2bit5/1 -> EL4xxx_0/6  "p32"
  [p_start] -> p_soll2bit9/2
  [p_start] -> p_soll2bit6/2
  p_soll2bit6/1 -> EL4xxx_0/7  "p41"
  [p_start] -> p_soll2bit8/2
  p_soll2bit8/1 -> EL4xxx_1/1  "p51"
  [p_start] -> p_soll2bit2/2
  p_soll2bit4/1 -> EL4xxx_0/5  "p31"
  p_soll2bit3/1 -> EL4xxx_0/4  "p22"
  MATLAB Function/4 -> Manual Switch3/1
  [p_start] -> p_soll2bit1/2
  p_soll2bit/1 -> EL4xxx_0/1  "p11"
  MATLAB Function/5 -> Manual Switch4/1
  p_soll2bit1/1 -> EL4xxx_0/2  "p12"
  p_soll2bit2/1 -> EL4xxx_0/3  "p21"
  [p_start] -> p_soll2bit7/2
  MATLAB Function/1 -> Manual Switch37/1
  p_start/1 -> [p_start]
  [p_start] -> p_soll2bit4/2
  MATLAB Function/9 -> Manual Switch8/1
  [p_start] -> p_soll2bit5/2
  [p_start] -> p_soll2bit/2
  MATLAB Function/8 -> Manual Switch7/1
  MATLAB Function/7 -> Manual Switch6/1
  MATLAB Function/2 -> Manual Switch1/1
  MATLAB Function/10 -> Manual Switch9/1
  MATLAB Function/6 -> Manual Switch5/1
  MATLAB Function/3 -> Manual Switch2/1
  p_d_bar/1 -> MATLAB Function/1
  Manual Switch37/1 -> p_soll2bit/1
  Manual Switch1/1 -> p_soll2bit1/1
  Manual Switch2/1 -> p_soll2bit2/1
  Manual Switch3/1 -> p_soll2bit3/1
  Manual Switch4/1 -> p_soll2bit4/1
  Manual Switch5/1 -> p_soll2bit5/1
  Manual Switch6/1 -> p_soll2bit6/1
  Manual Switch7/1 -> p_soll2bit7/1
  Manual Switch8/1 -> p_soll2bit8/1
  Constant11/1 -> Manual Switch37/2
  Constant13/1 -> Manual Switch1/2
  Constant2/1 -> Manual Switch2/2
  Constant3/1 -> Manual Switch3/2
  Constant14/1 -> Manual Switch4/2
  Constant15/1 -> Manual Switch5/2
  Constant6/1 -> Manual Switch6/2
  Constant7/1 -> Manual Switch7/2
  Constant8/1 -> Manual Switch8/2
  Constant9/1 -> Manual Switch9/2
  Manual Switch9/1 -> p_soll2bit9/1

== system test_bench/positions/Triggered Subsystem ==
  In1 : Inport
  Trigger : TriggerPort  VariantControl=Variant
  Out1 : Outport
  wires:
  In1/1 -> Out1/1

== system test_bench/positions/Triggered Subsystem1 ==
  In1 : Inport
  Trigger : TriggerPort  VariantControl=Variant
  Out1 : Outport
  wires:
  In1/1 -> Out1/1

== system test_bench/positions/Triggered Subsystem2 ==
  In1 : Inport
  Trigger : TriggerPort  VariantControl=Variant
  Out1 : Outport
  wires:
  In1/1 -> Out1/1

== system test_bench/positions/Triggered Subsystem3 ==
  In1 : Inport
  Trigger : TriggerPort  VariantControl=Variant
  Out1 : Outport
  wires:
  In1/1 -> Out1/1

== system test_bench/positions/Triggered Subsystem4 ==
  In1 : Inport
  Trigger : TriggerPort  VariantControl=Variant
  Out1 : Outport
  wires:
  In1/1 -> Out1/1

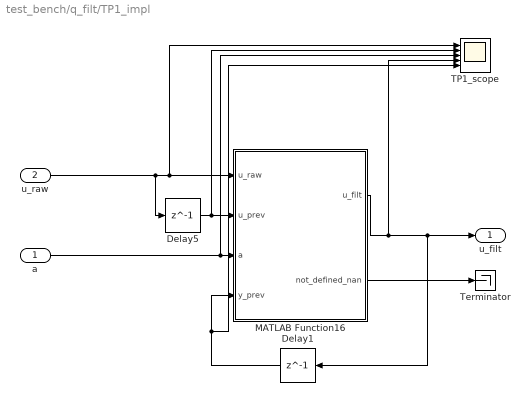
== system test_bench/q_filt/TP1_impl ==
  a : Inport
  u_raw : Inport  Port=2
  Delay1 : Delay  DelayLength=1  InitialCondition=zeros(1,5)  SampleTime=t_sample_s
  Delay5 : Delay  DelayLength=1  InitialCondition=zeros(1,5)  SampleTime=t_sample_s
  MATLAB Function16 : MATLAB Function  TreatAsAtomicUnit=on
  "TP1_scope " : Scope  NumInputPorts=5
  Terminator : Terminator
  u_filt : Outport  VectorParamsAs1DForOutWhenUnconnected=on
  wires:
  Delay5/1 -> "TP1_scope "/2, MATLAB Function16/2(u_prev)
  u_raw/1 -> Delay5/1, "TP1_scope "/1, MATLAB Function16/1(u_raw)
  MATLAB Function16/1(u_filt) -> "TP1_scope "/4, Delay1/1, u_filt/1
  a/1 -> "TP1_scope "/3, MATLAB Function16/3(a)
  Delay1/1 -> "TP1_scope "/5, MATLAB Function16/4(y_prev)
  MATLAB Function16/2(not_defined_nan) -> Terminator/1

== matlab function MATLAB Function ==
  data: idx input double; u input double; y output double
function y = fcn(idx, u)

y = squeeze(u(idx,:)');

== matlab function Subsystem4/MATLAB Function ==
  data: x input double; y output double; pred_horizon parameter double
function y = to1D(x,pred_horizon)
y = [pred_horizon,...
    x(:,1)',...
    x(:,2)',...
    x(:,3)',...
    x(:,4)',...
    x(:,5)'];

== matlab function q_filt/num diff ==
  data: q_deg input double; qd_degs output double; prev_q_deg input double; t_sample_s input double
function qd_degs = fcn(q_deg, prev_q_deg, t_sample_s)

qd_degs = (q_deg-prev_q_deg)/t_sample_s;

== matlab function subtract_offset ==
  data: q_deg_raw input double; q_deg_raw output double; q_offset input double
function q_deg_raw = subtract_offset(q_deg_raw,q_offset)

q_deg_raw = q_deg_raw-q_offset;

== matlab function MATLAB Function4 ==
  data: idx input double; u input double; y output double
function y = fcn(idx, u)

y = squeeze(u(idx,:)');

== matlab function Subsystem4/MATLAB Function1 ==
  data: x input double; y output double; pred_horizon parameter double
function y = to1D(x,pred_horizon)
y = [pred_horizon,...
    x(:,1)',...
    x(:,2)',...
    x(:,3)',...
    x(:,4)',...
    x(:,5)'];

== matlab function q_filt/TP1_impl/MATLAB Function16 ==
  data: u_raw input double; u_filt output double; u_prev input double; a input double; y_prev input double; not_defined_nan output double
function  [u_filt, not_defined_nan] = TP1_DiffEq_(u_raw, u_prev, a, y_prev)
if isnan(sum(u_raw))
    u_filt = zeros(5,1);
    not_defined_nan = 1;
elseif isnan(sum(TP1_DiffEq(u_raw, u_prev, a, y_prev)))
        u_filt = zeros(5,1);
        not_defined_nan = 2;
else
    u_filt = TP1_DiffEq(u_raw, u_prev, a, y_prev);
    not_defined_nan = 0;
end
